simulink model "Sim_Ex21"  (R2025a)
settings: Solver=FixedStepAuto  StartTime=0.0  StopTime=Stop_Time  FixedStep=step_time  RelTol=1e-3
values from neighbouring files (symbols this model uses):
  L = 1e-3    (= 0.001)    [A_Ex21.m]
  R = 1    [A_Ex21.m]
  Ts = 1/fs    (= 0.0002)    [A_Ex21.m]
  Tsw = 1/fsw    (= 0.0004)    [A_Ex21.m]
  V = 120    [A_Ex21.m]
  Vdc = 310    [A_Ex21.m]
  W = 2*pi*200    (= 1256.63706144)    [A_Ex21.m]
undefined symbols (not defined in the file or in its folder): DiscIntNeverNeededParam
libraries: simulink x1
settings Model: Creator=KYC  LastModifiedBy=moon
settings SolverCC: AlgebraicLoopSolver=TrustRegion
settings DataIOCC: ReturnWorkspaceOutputs=off
settings DebuggingCC: UnconnectedInputMsg=warning  UnconnectedOutputMsg=warning  UnconnectedLineMsg=warning  ArithmeticOperatorsInVariantConditions=warning
settings ModelReferenceCC: EnableRefExpFcnMdlSchedulingChecks=on
settings SFSimCC: SimUseLocalCustomCode=off  CustomCodeUndefinedFunction=UseInterfaceOnly
settings RTWCC: RTWUseLocalCustomCode=off  GPUComputeCapability=3.5
settings CodeAppCC: StateflowObjectComments=on

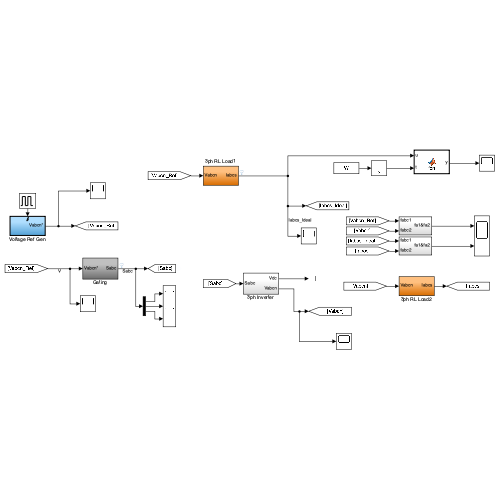
[thumbnail: Simulink's stored preview of the top-level diagram]
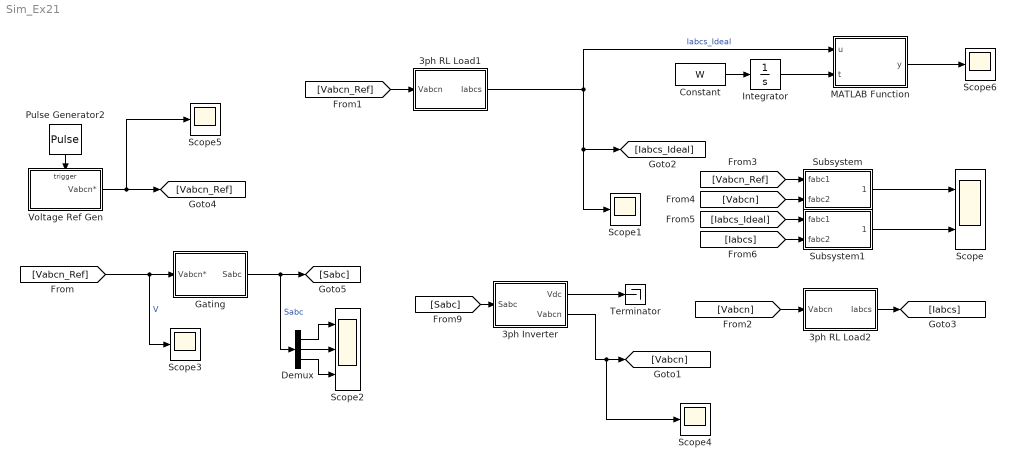
== system Sim_Ex21 ==
  3ph Inverter : Subsystem
  3ph RL Load1 : Subsystem
  3ph RL Load2 : Subsystem
  Constant : Constant  Value=W
  Demux : Demux  Outputs=3
  Gating : Subsystem
  Integrator : Integrator
  MATLAB Function : MATLAB Function  TreatAsAtomicUnit=on
  Pulse Generator2 : DiscretePulseGenerator  PulseType=Time based  Period=Ts  PulseWidth=50
  Scope : Scope  NumInputPorts=2
      settings: ActiveDisplayYMinimum=-258.33333  ActiveDisplayYMaximum=258.33333
  Scope{1,3..6} (5 alike) : Scope
      Scope1 settings: ActiveDisplayYMinimum=-1  ActiveDisplayYMaximum=1  DataLoggingVariableName=ScopeData3
      Scope3 settings: ActiveDisplayYMinimum=-1  ActiveDisplayYMaximum=1  DataLoggingVariableName=ScopeData5
      Scope4 settings: ActiveDisplayYMinimum=-193.75  ActiveDisplayYMaximum=193.75  DataLoggingVariableName=ScopeData6
      Scope5 settings: ActiveDisplayYMinimum=-1  ActiveDisplayYMaximum=1  DataLoggingVariableName=ScopeData7
      Scope6 settings: ActiveDisplayYMinimum=-193.75  ActiveDisplayYMaximum=193.75  DataLoggingVariableName=ScopeData10
  Scope2 : Scope  NumInputPorts=3
      settings: ActiveDisplayYMinimum=-1  ActiveDisplayYMaximum=1  DataLoggingVariableName=ScopeData4
  Subsystem : Subsystem
  Subsystem1 : Subsystem
  Terminator : Terminator
  Voltage Ref Gen : Subsystem
  wires:
  Pulse Generator2/1 -> Voltage Ref Gen/Trigger
  Voltage Ref Gen/1(Vabcn*) -> Scope5/1, [Vabcn_Ref]
  [Vabcn_Ref] -> Scope3/1, Gating/1(Vabcn*)  "V"
  3ph Inverter/2(Vabcn) -> Scope4/1, [Vabcn]
  [Vabcn] -> 3ph RL Load2/1(Vabcn)
  [Vabcn_Ref] -> 3ph RL Load1/1(Vabcn)
  3ph RL Load1/1(Iabcs) -> MATLAB Function/1(u), Scope1/1, [Iabcs_Ideal]  "Iabcs_Ideal"
  3ph RL Load2/1(Iabcs) -> [Iabcs]
  Subsystem/1(fa1&fa2) -> Scope/1
  Subsystem1/1(fa1&fa2) -> Scope/2
  [Vabcn_Ref] -> Subsystem/1(fabc1)
  [Vabcn] -> Subsystem/2(fabc2)
  [Iabcs_Ideal] -> Subsystem1/1(fabc1)
  [Iabcs] -> Subsystem1/2(fabc2)
  Gating/1(Sabc) -> Demux/1, [Sabc]  "Sabc"
  [Sabc] -> 3ph Inverter/1(Sabc)
  3ph Inverter/1(Vdc) -> Terminator/1
  Demux/1 -> Scope2/1
  Demux/2 -> Scope2/2
  Demux/3 -> Scope2/3
  MATLAB Function/1(y) -> Scope6/1
  Constant/1 -> Integrator/1
  Integrator/1 -> MATLAB Function/2(t)

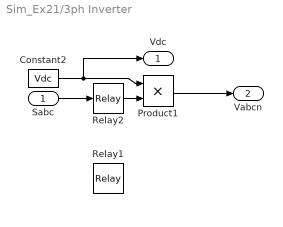
== system Sim_Ex21/3ph Inverter ==
  Sabc : Inport
  Constant2 : Constant  Value=Vdc
  Product1 : Product  RndMeth=Zero
  Relay1 : Relay  OnSwitchValue=0.5  OffSwitchValue=0.5  OnOutputValue=1/2  OffOutputValue=-1/2  OutDataTypeStr=double
  Relay2 : Relay  OnSwitchValue=0.5  OffSwitchValue=0.5  OnOutputValue=1/2  OffOutputValue=-1/2  OutDataTypeStr=double
  Vdc : Outport
  Vabcn : Outport  Port=2
  wires:
  Constant2/1 -> Vdc/1, Product1/1
  Sabc/1 -> Relay2/1
  Relay2/1 -> Product1/2
  Product1/1 -> Vabcn/1

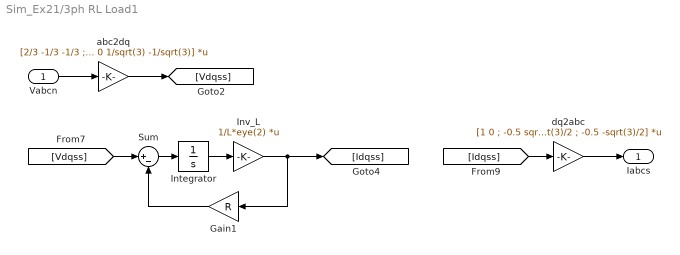
== system Sim_Ex21/3ph RL Load1 ==
  Vabcn : Inport
  Gain1 : Gain  Gain=R
  Integrator : Integrator
  Inv_L : Gain  Gain=1/L*eye(2)  Multiplication=Matrix(K*u)
  Sum : Sum  Inputs=|+-
  abc2dq : Gain  Gain=[2/3 -1/3 -1/3 ; 0 1/sqrt(3) -1/sqrt(3)]  Multiplication=Matrix(K*u)  SaturateOnIntegerOverflow=on  OutDataTypeStr=Inherit: Same as input  ParamDataTypeStr=Inherit: Same as input
  dq2abc : Gain  Gain=[1 0 ; -0.5 sqrt(3)/2 ; -0.5 -sqrt(3)/2]  Multiplication=Matrix(K*u)
  Iabcs : Outport
  wires:
  dq2abc/1 -> Iabcs/1
  [Idqss] -> dq2abc/1
  Inv_L/1 -> Gain1/1, [Idqss]
  Integrator/1 -> Inv_L/1
  [Vdqss] -> Sum/1
  Sum/1 -> Integrator/1
  Gain1/1 -> Sum/2
  Vabcn/1 -> abc2dq/1
  abc2dq/1 -> [Vdqss]

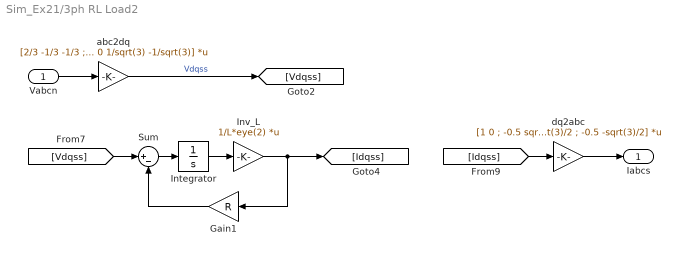
== system Sim_Ex21/3ph RL Load2 ==
  Vabcn : Inport
  Gain1 : Gain  Gain=R
  Integrator : Integrator
  Inv_L : Gain  Gain=1/L*eye(2)  Multiplication=Matrix(K*u)
  Sum : Sum  Inputs=|+-
  abc2dq : Gain  Gain=[2/3 -1/3 -1/3 ; 0 1/sqrt(3) -1/sqrt(3)]  Multiplication=Matrix(K*u)  SaturateOnIntegerOverflow=on  OutDataTypeStr=Inherit: Same as input  ParamDataTypeStr=Inherit: Same as input
  dq2abc : Gain  Gain=[1 0 ; -0.5 sqrt(3)/2 ; -0.5 -sqrt(3)/2]  Multiplication=Matrix(K*u)
  Iabcs : Outport
  wires:
  abc2dq/1 -> [Vdqss]  "Vdqss"
  Vabcn/1 -> abc2dq/1
  Gain1/1 -> Sum/2
  Sum/1 -> Integrator/1
  [Vdqss] -> Sum/1
  Integrator/1 -> Inv_L/1
  Inv_L/1 -> [Idqss], Gain1/1
  [Idqss] -> dq2abc/1
  dq2abc/1 -> Iabcs/1

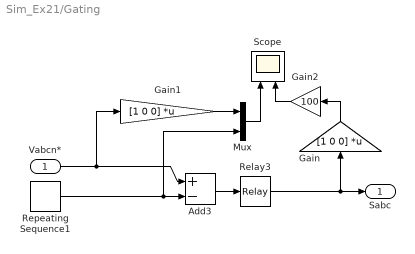
== system Sim_Ex21/Gating ==
  Vabcn* : Inport
  Add3 : Sum  Inputs=+-
  Gain : Gain  Gain=[1 0 0]  Multiplication=Matrix(K*u)
  Gain1 : Gain  Gain=[1 0 0]  Multiplication=Matrix(K*u)
  Gain2 : Gain  Gain=100
  Mux : Mux  Inputs=2
  Relay3 : Relay  OnSwitchValue=0  OffSwitchValue=0  OutDataTypeStr=double
  Repeating Sequence1 : simulink/Sources/Repeating Sequence  rep_seq_t=[0 Tsw/2 Tsw]  rep_seq_y=Vdc*[-0.5 0.5 0-0.5]
  Scope : Scope  NumInputPorts=2
      settings: ActiveDisplayYMinimum=-193.75  ActiveDisplayYMaximum=193.75  DataLoggingVariableName=ScopeData2
  Sabc : Outport
  wires:
  Add3/1 -> Relay3/1
  Vabcn*/1 -> Add3/1, Gain1/1
  Relay3/1 -> Gain/1, Sabc/1
  Mux/1 -> Scope/1
  Gain/1 -> Gain2/1
  Gain1/1 -> Mux/1
  Repeating Sequence1/1 -> Mux/2, Add3/2
  Gain2/1 -> Scope/2

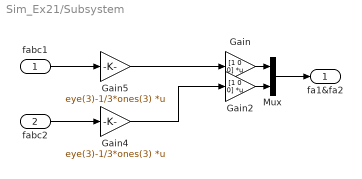
== system Sim_Ex21/Subsystem ==
  fabc1 : Inport
  fabc2 : Inport  Port=2
  Gain : Gain  Gain=[1 0 0]  Multiplication=Matrix(K*u)
  Gain2 : Gain  Gain=[1 0 0]  Multiplication=Matrix(K*u)
  Gain4 : Gain  Gain=eye(3)-1/3*ones(3)  Multiplication=Matrix(K*u)
  Gain5 : Gain  Gain=eye(3)-1/3*ones(3)  Multiplication=Matrix(K*u)
  Mux : Mux  Inputs=2
  fa1&fa2 : Outport
  wires:
  fabc2/1 -> Gain4/1
  fabc1/1 -> Gain5/1
  Gain5/1 -> Gain/1
  Mux/1 -> fa1&fa2/1
  Gain4/1 -> Gain2/1
  Gain2/1 -> Mux/2
  Gain/1 -> Mux/1

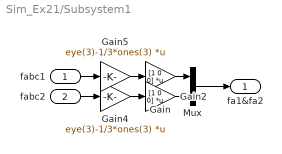
== system Sim_Ex21/Subsystem1 ==
  fabc1 : Inport
  fabc2 : Inport  Port=2
  Gain : Gain  Gain=[1 0 0]  Multiplication=Matrix(K*u)
  Gain2 : Gain  Gain=[1 0 0]  Multiplication=Matrix(K*u)
  Gain4 : Gain  Gain=eye(3)-1/3*ones(3)  Multiplication=Matrix(K*u)
  Gain5 : Gain  Gain=eye(3)-1/3*ones(3)  Multiplication=Matrix(K*u)
  Mux : Mux  Inputs=2
  fa1&fa2 : Outport
  wires:
  Gain/1 -> Mux/1
  Gain2/1 -> Mux/2
  Gain4/1 -> Gain2/1
  Mux/1 -> fa1&fa2/1
  Gain5/1 -> Gain/1
  fabc1/1 -> Gain5/1
  fabc2/1 -> Gain4/1

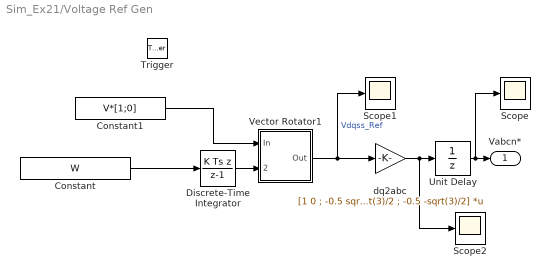
== system Sim_Ex21/Voltage Ref Gen ==
  Trigger : TriggerPort  VariantControl=Variant  PortDimensions=1
  Constant : Constant  Value=W
  Constant1 : Constant  Value=V*[1;0]
  Discrete-Time Integrator : DiscreteIntegrator  IntegratorMethod=Integration: Backward Euler  SampleTime=-1  ICPrevOutput=DiscIntNeverNeededParam  ICPrevScaledInput=DiscIntNeverNeededParam
  Scope : Scope
      settings: ActiveDisplayYMinimum=-1  ActiveDisplayYMaximum=1
  Scope1 : Scope
      settings: ActiveDisplayYMinimum=-242.1875  ActiveDisplayYMaximum=242.1875  DataLoggingVariableName=ScopeData8
  Scope2 : Scope
      settings: ActiveDisplayYMinimum=-1  ActiveDisplayYMaximum=1  DataLoggingVariableName=ScopeData9
  Unit Delay : UnitDelay  SampleTime=-1  HasFrameUpgradeWarning=on
  Vector Rotator1 : Subsystem
  dq2abc : Gain  Gain=[1 0 ; -0.5 sqrt(3)/2 ; -0.5 -sqrt(3)/2]  Multiplication=Matrix(K*u)
  Vabcn* : Outport  InitialOutput=[0]
  wires:
  dq2abc/1 -> Scope2/1, Unit Delay/1
  Constant/1 -> Discrete-Time Integrator/1
  Discrete-Time Integrator/1 -> Vector Rotator1/2(Theta)
  Constant1/1 -> Vector Rotator1/1(In)
  Vector Rotator1/1(Out) -> Scope1/1, dq2abc/1  "Vdqss_Ref"
  Unit Delay/1 -> Scope/1, Vabcn*/1

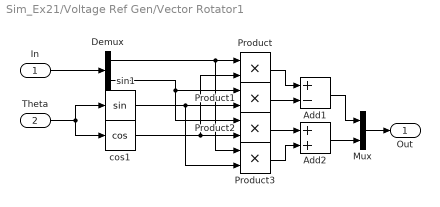
== system Sim_Ex21/Voltage Ref Gen/Vector Rotator1 ==
  In : Inport
  Theta : Inport  Port=2
  Add1 : Sum  Inputs=+-
  Add2 : Sum
  Demux : Demux  Outputs=2
  Mux : Mux  Inputs=[1 1]
  Product{,1..3} (4 alike) : Product  RndMeth=Zero
  cos1 : Trigonometry  Operator=cos
  sin1 : Trigonometry
  Out : Outport
  wires:
  Theta/1 -> cos1/1, sin1/1
  Demux/1 -> Product3/1, Product/1
  Mux/1 -> Out/1
  In/1 -> Demux/1
  Demux/2 -> Product1/1, Product2/1
  cos1/1 -> Product/2, Product2/2
  sin1/1 -> Product1/2, Product3/2
  Product/1 -> Add1/1
  Product1/1 -> Add1/2
  Add1/1 -> Mux/1
  Product2/1 -> Add2/1
  Product3/1 -> Add2/2
  Add2/1 -> Mux/2

== matlab function Sim_Ex21/MATLAB Function ==
  data: u input; y output; t input
function y = fcn(u, t)
a=2*pi/3;
T = [cos(t)  cos(t-a)  cos(t+a);
    -sin(t) -sin(t-a) -sin(t+a);] * 2/3;

y = T*u;
